simulink model "DcMotorPositionControlSimulink"  (R2019b)
settings: Solver=VariableStepAuto  StartTime=0.0  StopTime=0.2  RelTol=1e-3
values from neighbouring files (symbols this model uses):
  b = 0.1    [DcMotorSpeedControl.m]
  J = 0.01    [DcMotorSpeedControl.m]
  K = 0.01    [DcMotorSpeedControl.m]
  L = 0.5    [DcMotorSpeedControl.m]
  R = 1    [DcMotorSpeedControl.m]
settings Model: Creator=fhasan1  LastModifiedBy=fhasan1

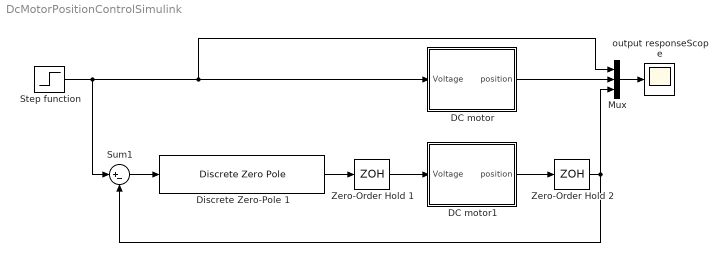
== system DcMotorPositionControlSimulink ==
  DC motor : Subsystem
  DC motor1 : Subsystem
  Discrete Zero-Pole 1 : DiscreteZeroPole  Zeros=[0.95 0.8 0.8]  Poles=[-0.98 0.6 1]  Gain=800  SampleTime=-1
  Mux : Mux  Inputs=3
  Step function : Step  Time=0  SampleTime=0
  Sum1 : Sum  Inputs=|+-
  Zero-Order Hold 1 : ZeroOrderHold  SampleTime=0.001
  Zero-Order Hold 2 : ZeroOrderHold  SampleTime=0.001
  "output responseScope " : Scope
  wires:
  DC motor/1(position) -> Mux/2
  Mux/1 -> "output responseScope "/1
  Step function/1 -> Mux/1, DC motor/1(Voltage), Sum1/1
  Discrete Zero-Pole 1/1 -> Zero-Order Hold 1/1
  Zero-Order Hold 1/1 -> DC motor1/1(Voltage)
  Sum1/1 -> Discrete Zero-Pole 1/1
  DC motor1/1(position) -> Zero-Order Hold 2/1
  Zero-Order Hold 2/1 -> Sum1/2, Mux/3

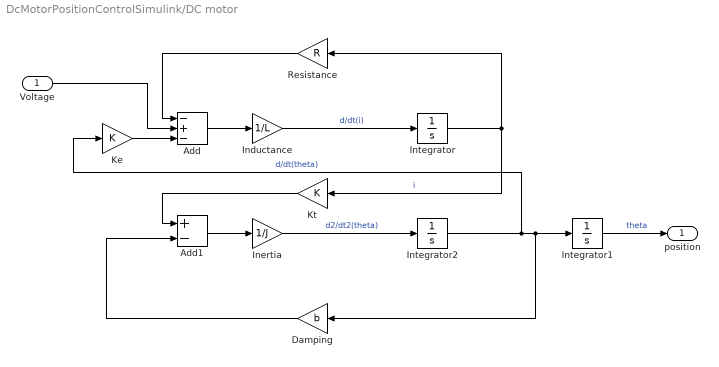
== system DcMotorPositionControlSimulink/DC motor ==
  Voltage : Inport
  Add : Sum  Inputs=-+-
  Add1 : Sum  Inputs=+-
  Damping : Gain  Gain=b
  Inductance : Gain  Gain=1/L
  Inertia : Gain  Gain=1/J
  Integrator : Integrator
  Integrator1 : Integrator
  Integrator2 : Integrator
  Ke : Gain  Gain=K
  Kt : Gain  Gain=K
  Resistance : Gain  Gain=R
  position : Outport
  wires:
  Integrator2/1 -> Ke/1, Integrator1/1, Damping/1  "d/dt(theta)"
  Add/1 -> Inductance/1
  Kt/1 -> Add1/1
  Damping/1 -> Add1/2
  Add1/1 -> Inertia/1
  Integrator/1 -> Resistance/1, Kt/1  "i"
  Inductance/1 -> Integrator/1  "d/dt(i)"
  Resistance/1 -> Add/1
  Inertia/1 -> Integrator2/1  "d2/dt2(theta)"
  Voltage/1 -> Add/2
  Ke/1 -> Add/3
  Integrator1/1 -> position/1  "theta"

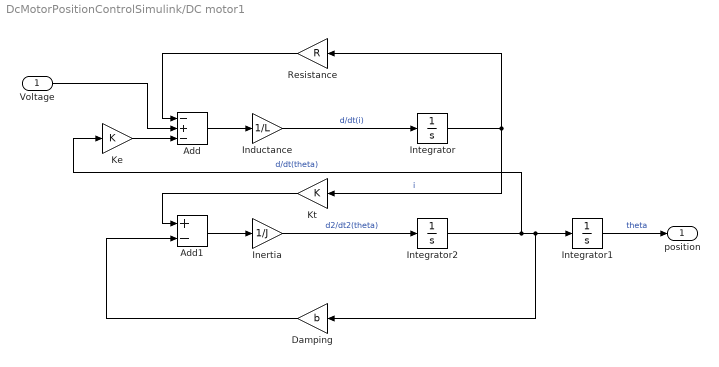
== system DcMotorPositionControlSimulink/DC motor1 ==
  Voltage : Inport
  Add : Sum  Inputs=-+-
  Add1 : Sum  Inputs=+-
  Damping : Gain  Gain=b
  Inductance : Gain  Gain=1/L
  Inertia : Gain  Gain=1/J
  Integrator : Integrator
  Integrator1 : Integrator
  Integrator2 : Integrator
  Ke : Gain  Gain=K
  Kt : Gain  Gain=K
  Resistance : Gain  Gain=R
  position : Outport
  wires:
  Integrator2/1 -> Ke/1, Integrator1/1, Damping/1  "d/dt(theta)"
  Add/1 -> Inductance/1
  Kt/1 -> Add1/1
  Damping/1 -> Add1/2
  Add1/1 -> Inertia/1
  Integrator/1 -> Resistance/1, Kt/1  "i"
  Inductance/1 -> Integrator/1  "d/dt(i)"
  Resistance/1 -> Add/1
  Inertia/1 -> Integrator2/1  "d2/dt2(theta)"
  Voltage/1 -> Add/2
  Ke/1 -> Add/3
  Integrator1/1 -> position/1  "theta"
